simulink model "Blank_SS_ABCD"  (R2018b)
settings: Solver=VariableStepAuto  StartTime=0.0  StopTime=10.0  RelTol=1e-3
undefined symbols (not defined in the file): As, Bs, Cs, Ds
settings Model: Creator=Johan PC  LastModifiedBy=Johan PC

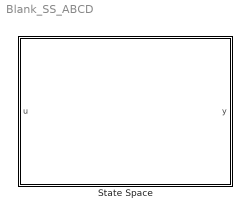
== system Blank_SS_ABCD ==
  State Space : Subsystem

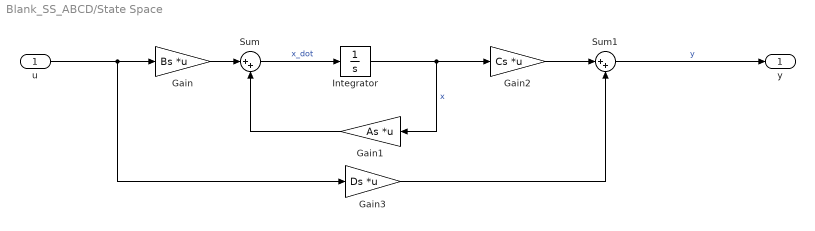
== system Blank_SS_ABCD/State Space ==
  u : Inport
  Gain : Gain  Gain=Bs  Multiplication=Matrix(K*u)
  Gain1 : Gain  Gain=As  Multiplication=Matrix(K*u)
  Gain2 : Gain  Gain=Cs  Multiplication=Matrix(K*u)
  Gain3 : Gain  Gain=Ds  Multiplication=Matrix(K*u)
  Integrator : Integrator
  Sum : Sum  Inputs=|++
  Sum1 : Sum  Inputs=|++
  y : Outport
  wires:
  Sum1/1 -> y/1  "y"
  Gain/1 -> Sum/1
  Integrator/1 -> Gain1/1, Gain2/1  "x"
  Gain2/1 -> Sum1/1
  u/1 -> Gain3/1, Gain/1
  Sum/1 -> Integrator/1  "x_dot"
  Gain3/1 -> Sum1/2
  Gain1/1 -> Sum/2
